simulink model "tcm_nobus"  (Simulink 8.5)
settings: Solver=ode3  StartTime=0.0  StopTime=10.0  RelTol=1e-3
undefined symbols (not defined in the file or in its folder): ap, bias, sgn
libraries: simulink x3
(part 2 of 2)

== system tcm_nobus/TCM/Longitudinal/Altitude Control/Variable  Rate Limit/Variable Limit Saturation ==
  up_lim : Inport  RequirementInfo={} %GIDa_c3426702_ae57_4a6b_8e5b_d8e7ea7997b8
  SigIn : Inport  RequirementInfo={} %GIDa_57ffe4bd_514b_4f1d_925b_ea07d6710330  Port=2
  Lo_lim : Inport  RequirementInfo={} %GIDa_934c3ebb_c2a8_4cb2_b1d4_7a7b38287908  Port=3
  Enforce low lim : MinMax  RequirementInfo={} %GIDa_f320f771_b833_4e25_ab12_e91693dd9b04  Function=max  Inputs=2
  Enforce up lim : MinMax  RequirementInfo={} %GIDa_1cfdde9a_faa1_4e7e_9516_cacb3f0cb773  Inputs=2
  Out1 : Outport  RequirementInfo={} %GIDa_6b324e36_3b21_43eb_ae92_bdd39356922a
  wires:
  Enforce up lim/1 -> Out1/1
  up_lim/1 -> Enforce up lim/2
  Enforce low lim/1 -> Enforce up lim/1
  SigIn/1 -> Enforce low lim/2
  Lo_lim/1 -> Enforce low lim/1
